simulink model "V_f_cdinamico_MPC"  (R2021b)
settings: Solver=VariableStepAuto  StartTime=0.0  StopTime=110  RelTol=1e-3
libraries: dsparch4 x3, mpclib x1, simulink x1
settings Model: Creator=Braulio  LastModifiedBy=bmr

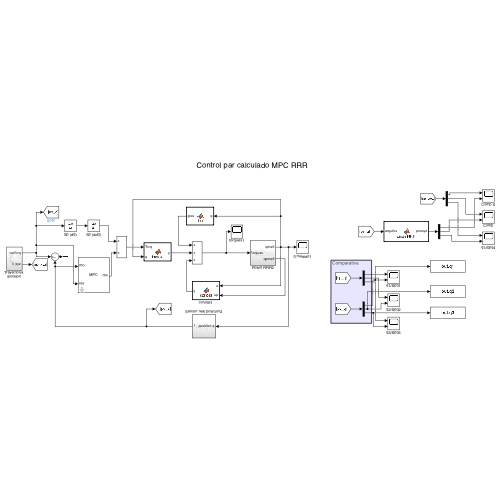
[thumbnail: Simulink's stored preview of the top-level diagram]
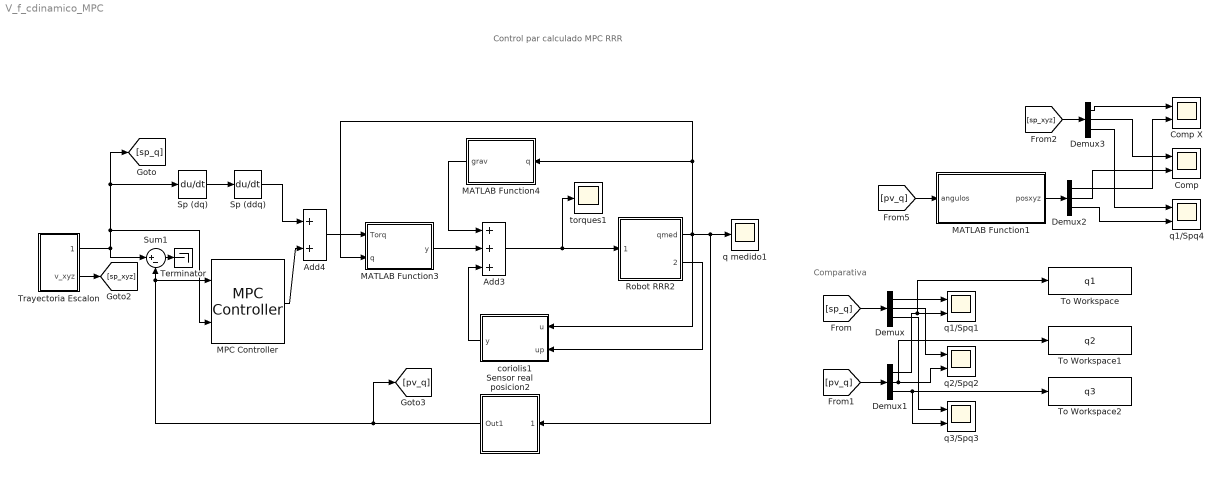
== system V_f_cdinamico_MPC ==
  note: Control par calculado MPC RRR
  note: Comparativa
  Add3 : Sum  Inputs=+++
  Add4 : Sum
  Comp : Scope  NumInputPorts=2
  Comp X : Scope  NumInputPorts=2
  Demux{,1..3} (4 alike) : Demux  Outputs=3
  MATLAB Function1 : MATLAB Function  TreatAsAtomicUnit=on
  MATLAB Function3 : MATLAB Function  TreatAsAtomicUnit=on
  MATLAB Function4 : MATLAB Function  TreatAsAtomicUnit=on
  MPC Controller : mpclib/MPC Controller  SCDEnableBlockLinearizationSpecification=on  mpcobj=mpc1  is_multiple=0  enable_value=0  return_u0=off  updateMPCinCallerWorkspace=on  md_inport=off  mv_inport=off  uref_inport=off  return_cost=off  return_mvseq=off  return_qpstatus=off  return_xseq=off  return_state=off  return_ovseq=off  state_inport=off  umin_inport=off  umax_inport=off  ymin_inport=off  ymax_inport=off  cc_inport=off  ywt_inport=off  uwt_inport=off  duwt_inport=off  rhoeps_inport=off  pm_inport=off  MaximumP=10  HorizonChoice=FixedHorizon  n_ts=0.1  n_p=10  n_mv=3  n_md=0  n_ud=0  n_mo=3  n_uo=0  BlockDataType=double  SampleTimeInherited=off  switch_inport=off
  Robot RRR2 : Subsystem
  Sensor real posicion2 : Subsystem
  Sp (ddq) : Derivative
  Sp (dq) : Derivative
  Sum1 : Sum  Inputs=|+-
  Terminator : Terminator
  To Workspace : ToWorkspace  VariableName=q1  SampleTime=0.1
  To Workspace1 : ToWorkspace  VariableName=q2  SampleTime=0.1
  To Workspace2 : ToWorkspace  VariableName=q3  SampleTime=0.1
  Trayectoria Escalon : Subsystem
  coriolis1 : MATLAB Function  TreatAsAtomicUnit=on
  q medido1 : Scope
  q1/Spq1 : Scope  NumInputPorts=2
  q1/Spq4 : Scope  NumInputPorts=2
  q2/Spq2 : Scope  NumInputPorts=2
  q3/Spq3 : Scope  NumInputPorts=2
  torques1 : Scope
  wires:
  MPC Controller/1 -> Add4/2
  Sp (ddq)/1 -> Add4/1
  Trayectoria Escalon/1(vectorq) -> MPC Controller/2, [sp_q], Sp (dq)/1, Sum1/1
  MATLAB Function4/1(grav) -> Add3/1
  Sp (dq)/1 -> Sp (ddq)/1
  MATLAB Function3/1(y) -> Add3/2
  Sensor real posicion2/1(Out1) -> [pv_q], MPC Controller/1, Sum1/2
  Trayectoria Escalon/2(v_xyz) -> [sp_xyz]
  Add4/1 -> MATLAB Function3/1(Torq)
  [sp_xyz] -> Demux3/1
  Demux/3 -> q3/Spq3/1
  Demux3/1 -> Comp X/1
  MATLAB Function1/1(posxyz) -> Demux2/1
  [pv_q] -> Demux1/1
  Demux2/1 -> Comp X/2
  Demux3/2 -> Comp/1
  Demux2/3 -> q1/Spq4/2
  Demux1/3 -> q3/Spq3/2, To Workspace2/1
  Add3/1 -> Robot RRR2/1(torques), torques1/1
  Demux1/1 -> To Workspace/1, q1/Spq1/2
  Demux1/2 -> q2/Spq2/2, To Workspace1/1
  Demux3/3 -> q1/Spq4/1
  coriolis1/1(y) -> Add3/3
  Demux2/2 -> Comp/2
  [sp_q] -> Demux/1
  Demux/1 -> q1/Spq1/1
  Demux/2 -> q2/Spq2/1
  Robot RRR2/1(qmed) -> q medido1/1, Sensor real posicion2/1(posicion q), coriolis1/1(u), MATLAB Function3/2(q), MATLAB Function4/1(q)
  Robot RRR2/2(qpmed) -> coriolis1/2(up)
  [pv_q] -> MATLAB Function1/1(angulos)
  Sum1/1 -> Terminator/1

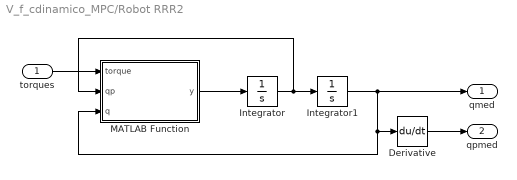
== system V_f_cdinamico_MPC/Robot RRR2 ==
  torques : Inport
  Derivative : Derivative
  Integrator : Integrator
  Integrator1 : Integrator  LimitOutput=on  UpperSaturationLimit=1.39626  LowerSaturationLimit=-1.39626
  MATLAB Function : MATLAB Function  TreatAsAtomicUnit=on
  qmed : Outport
  qpmed : Outport  Port=2
  wires:
  Integrator1/1 -> qmed/1, MATLAB Function/3(q), Derivative/1
  MATLAB Function/1(y) -> Integrator/1
  Integrator/1 -> MATLAB Function/2(qp), Integrator1/1
  torques/1 -> MATLAB Function/1(torque)
  Derivative/1 -> qpmed/1

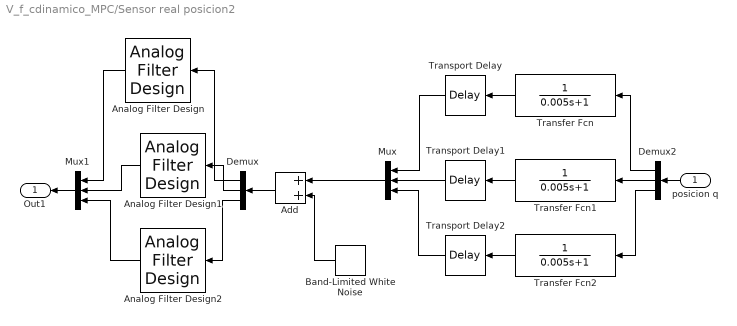
== system V_f_cdinamico_MPC/Sensor real posicion2 ==
  posicion q : Inport
  Add : Sum
  Analog Filter Design : dsparch4/Analog Filter Design  method=Butterworth  filttype=Lowpass  N=8  Wlo=30  Whi=80  Rp=2  Rs=40
  Analog Filter Design1 : dsparch4/Analog Filter Design  method=Butterworth  filttype=Lowpass  N=8  Wlo=30  Whi=80  Rp=2  Rs=40
  Analog Filter Design2 : dsparch4/Analog Filter Design  method=Butterworth  filttype=Lowpass  N=8  Wlo=30  Whi=80  Rp=2  Rs=40
  Band-Limited White Noise : simulink/Sources/Band-Limited White Noise  Cov=[0.00001]  Ts=0.1  seed=[23341]
  Demux : Demux  Outputs=3
  Demux2 : Demux  Outputs=3
  Mux : Mux  Inputs=3
  Mux1 : Mux  Inputs=3
  Transfer Fcn : TransferFcn  Denominator=[0.005 1]
  Transfer Fcn1 : TransferFcn  Denominator=[0.005 1]
  Transfer Fcn2 : TransferFcn  Denominator=[0.005 1]
  Transport Delay : TransportDelay  DelayTime=0.05
  Transport Delay1 : TransportDelay  DelayTime=0.05
  Transport Delay2 : TransportDelay  DelayTime=0.05
  Out1 : Outport
  wires:
  Analog Filter Design2/1 -> Mux1/3
  Analog Filter Design1/1 -> Mux1/2
  Analog Filter Design/1 -> Mux1/1
  Mux1/1 -> Out1/1
  Demux/3 -> Analog Filter Design2/1
  Demux/2 -> Analog Filter Design1/1
  Demux/1 -> Analog Filter Design/1
  Add/1 -> Demux/1
  Mux/1 -> Add/1
  Band-Limited White Noise/1 -> Add/2
  posicion q/1 -> Demux2/1
  Demux2/1 -> Transfer Fcn/1
  Transport Delay2/1 -> Mux/3
  Transport Delay1/1 -> Mux/2
  Transfer Fcn2/1 -> Transport Delay2/1
  Transport Delay/1 -> Mux/1
  Demux2/2 -> Transfer Fcn1/1
  Transfer Fcn/1 -> Transport Delay/1
  Demux2/3 -> Transfer Fcn2/1
  Transfer Fcn1/1 -> Transport Delay1/1

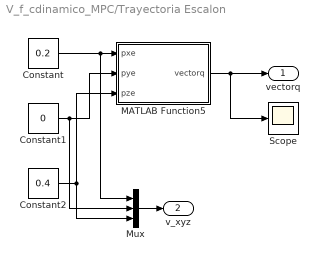
== system V_f_cdinamico_MPC/Trayectoria Escalon ==
  Constant : Constant  Value=0.2
  Constant1 : Constant  Value=0
  Constant2 : Constant  Value=0.4
  MATLAB Function5 : MATLAB Function  TreatAsAtomicUnit=on
  Mux : Mux  Inputs=3
  Scope : Scope
  vectorq : Outport
  v_xyz : Outport  Port=2
  wires:
  Constant1/1 -> Mux/2, MATLAB Function5/2(pye)
  Constant/1 -> Mux/1, MATLAB Function5/1(pxe)
  Constant2/1 -> MATLAB Function5/3(pze), Mux/3
  MATLAB Function5/1(vectorq) -> Scope/1, vectorq/1
  Mux/1 -> v_xyz/1

== matlab function V_f_cdinamico_MPC/MATLAB Function1 ==
  data: angulos input size=3; posxyz output size=3
%% Funcion cinematica directa
function posxyz = cindinRRR(angulos)
%% Vector angulo de 3 dim.
th1=angulos(1);
th2=angulos(2);
th3=angulos(3);
%% Valores eslabones
L1=0.2;L2=0.2;L3=0.2;
%% pos
xe=cos(th1)*(L3*cos(th2+th3) + L2*cos(th2));
ye=sin(th1)*(L3*cos(th2+th3) + L2*cos(th2));
ze=L1+(L3*sin(th2+th3)) +L2*sin(th2);
posxyz=[xe;ye;ze];

== matlab function V_f_cdinamico_MPC/MATLAB Function3 ==
  data: Torq input; y output; q input
function y = inercia(Torq, q)

tau1c=Torq(1);
tau2c=Torq(2);
tau3c=Torq(3);
th1=q(1);
th2=q(2);
th3=q(3);

Tauc=[tau1c;
      tau2c;
      tau3c];

L1=1;
L2=1;
L3=1;
m1=1;
m2=1;
m3=1;
g=9.81;

M11=(L2^2*m2)/8 + (L2^2*m3)/2 + (L3^2*m3)/8 + (L2^2*m2*cos(2*th2))/8 + (L2^2*m3*cos(2*th2))/2 + (L3^2*m3*cos(2*th2 + 2*th3))/8 + (L2*L3*m3*cos(th3))/2 + (L2*L3*m3*cos(2*th2 + th3))/2;
M12=0;
M13=0;

M21=0;
M22=(L2^2*m2)/4 + L2^2*m3 + (L3^2*m3)/4 + L2*L3*m3*cos(th3);
M23=(L3*m3*(L3 + 2*L2*cos(th3)))/4;

M31=0;
M32=(L3*m3*(L3/2 + L2*cos(th3)))/2;
M33=(L3^2*m3)/4;

M=[M11 M12 M13;
    M21 M22 M23;
    M31 M32 M33];

y = M*Tauc;

== matlab function V_f_cdinamico_MPC/MATLAB Function4 ==
  data: q input size=3; grav output size=3
function grav = fcn(q)

th1 = q(1);
th2 = q(2);
th3 = q(3);


g = 9.81;
L1=0.2;
L2=0.2;
L3=0.2;

m1=1;
m2=1;
m3=1;
g=9.81;


g1=0;
g2=(L3*m3*cos(th2 + th3))/2 + (L2*m2*cos(th2))/2 + L2*m3*cos(th2);
g3=(L3*m3*cos(th2 + th3))/2;

grav = g*[g1;
          g2;
          g3];

== matlab function V_f_cdinamico_MPC/Robot RRR2/MATLAB Function ==
  data: torque input size=3; y output size=3; qp input size=3; q input size=3
function y = din_inv(torque, qp,q)

tau1 = torque(1);
tau2 = torque(2);
tau3 = torque(3);

th1=q(1);
th2=q(2);
th3=q(3);

th1p = qp(1);
th2p = qp(2);
th3p = qp(3);

Tau=[tau1;
     tau2;
     tau3];

L1=0.2;
L2=0.2;
L3=0.2;

m1=1;
m2=1;
m3=1;

g=9.81;

M11=(L2^2*m2)/8 + (L2^2*m3)/2 + (L3^2*m3)/8 + (L2^2*m2*cos(2*th2))/8 + (L2^2*m3*cos(2*th2))/2 + (L3^2*m3*cos(2*th2 + 2*th3))/8 + (L2*L3*m3*cos(th3))/2 + (L2*L3*m3*cos(2*th2 + th3))/2;
M12=0;
M13=0;

M21=0;
M22=(L2^2*m2)/4 + L2^2*m3 + (L3^2*m3)/4 + L2*L3*m3*cos(th3);
M23=(L3*m3*(L3 + 2*L2*cos(th3)))/4;

M31=0;
M32=(L3*m3*(L3/2 + L2*cos(th3)))/2;
M33=(L3^2*m3)/4;

M=[M11 M12 M13;
    M21 M22 M23;
    M31 M32 M33];



g1=0;
g2=(L3*m3*cos(th2 + th3))/2 + (L2*m2*cos(th2))/2 + L2*m3*cos(th2);
g3=(L3*m3*cos(th2 + th3))/2;

G=[g1;
   g2;
   g3];

b1=0.5;
b2=0.5;
b3=0.5;

F=[b1*th1p;
   b2*th2p;
   b3*th3p];

C1=-(th1p*(L3^2*m3*th2p*sin(th2 + 2*th3) + L3^2*m3*th3p*sin(2*th2 + th3) + L2^2*m2*th2p*sin(2*th2) + 4*L2^2*m3*th2p*sin(2*th2) + L3^2*m3*th2p*sin(2*th2 + 2*th3) + L3^2*m3*th3p*sin(2*th2 + 2*th3) - L3^2*m3*th2p*sin(th2) - L3^2*m3*th3p*sin(th3) + 2*L2*L3*m3*th3p*sin(2*th2) + 2*L2*L3*m3*th2p*sin(th2 + th3) + 2*L2*L3*m3*th3p*sin(th3) - 2*L2*L3*m3*th2p*sin(th2 - th3) + 4*L2*L3*m3*th2p*sin(2*th2 + th3) + 2*L2*L3*m3*th3p*sin(2*th2 + th3)))/8;
C2=(L2^2*m2*th1p^2*sin(2*th2))/8 + (L2^2*m3*th1p^2*sin(2*th2))/2 + (L3^2*m3*th1p^2*sin(2*th2 + 2*th3))/8 - (L2*L3*m3*th3p^2*sin(th3))/2 + (L2*L3*m3*th1p^2*sin(2*th2 + th3))/2 - L2*L3*m3*th2p*th3p*sin(th3);
C3=(L3*m3*(2*L2*th1p^2*sin(th3) + 4*L2*th2p^2*sin(th3) + 2*L2*th1p^2*sin(2*th2 + th3) + L3*th1p^2*sin(2*th2 + 2*th3)))/8;

C=[C1;
   C2;
   C3];

thpp=inv(M)*(Tau-C-F-(G*g));

y=thpp;

== matlab function V_f_cdinamico_MPC/coriolis1 ==
  data: u input size=3; y output size=3; up input
function y = coriolis(u,up)

th1=u(1);
th2=u(2);
th3=u(3);

th1p=up(1);
th2p=up(2);
th3p=up(3);

L1=0.2;
L2=0.2;
L3=0.2;
m1=1;
m2=1;
m3=1;
g=9.81;

C1=-(th1p*(L3^2*m3*th2p*sin(th2 + 2*th3) + L3^2*m3*th3p*sin(2*th2 + th3) + L2^2*m2*th2p*sin(2*th2) + 4*L2^2*m3*th2p*sin(2*th2) + L3^2*m3*th2p*sin(2*th2 + 2*th3) + L3^2*m3*th3p*sin(2*th2 + 2*th3) - L3^2*m3*th2p*sin(th2) - L3^2*m3*th3p*sin(th3) + 2*L2*L3*m3*th3p*sin(2*th2) + 2*L2*L3*m3*th2p*sin(th2 + th3) + 2*L2*L3*m3*th3p*sin(th3) - 2*L2*L3*m3*th2p*sin(th2 - th3) + 4*L2*L3*m3*th2p*sin(2*th2 + th3) + 2*L2*L3*m3*th3p*sin(2*th2 + th3)))/8;
C2=(L2^2*m2*th1p^2*sin(2*th2))/8 + (L2^2*m3*th1p^2*sin(2*th2))/2 + (L3^2*m3*th1p^2*sin(2*th2 + 2*th3))/8 - (L2*L3*m3*th3p^2*sin(th3))/2 + (L2*L3*m3*th1p^2*sin(2*th2 + th3))/2 - L2*L3*m3*th2p*th3p*sin(th3);
C3=(L3*m3*(2*L2*th1p^2*sin(th3) + 4*L2*th2p^2*sin(th3) + 2*L2*th1p^2*sin(2*th2 + th3) + L3*th1p^2*sin(2*th2 + 2*th3)))/8;

C=[C1;
   C2;
   C3];

y=C;

== matlab function V_f_cdinamico_MPC/Trayectoria Escalon/MATLAB Function5 ==
  data: pxe input size=1; vectorq output size=3; pye input size=1; pze input size=1
function vectorq = cininvRRR(pxe,pye,pze)
%% Valores 
L1=0.2;L2=0.2;L3=0.2;
%% angulos
q1=atan2(pye,pxe);
cq3=(pxe^2 +pye^2 +pze^2 -L2^2 -L3^2)/(2*L2*L3);
%% Condicionante para la variable cq3
if (cq3>=1)
    cq3=1;
end 

q3=atan2(sqrt(1-cq3),cq3);
beta=atan2(pze,sqrt(pxe^2 +pye^2));
alfa=atan2(L3*sin(q3),L2 +L3*cq3);
q2=beta-alfa;
vectorq=[q1;q2;q3];
